simulink model "factMatWhile"  (R2016b)
settings: Solver=FixedStepDiscrete  StartTime=0.0  StopTime=10.0  RelTol=1e-3
libraries: simulink x1
settings Model: Creator=Radwa  LastModifiedBy=Radwa
settings SolverCC: EnableConcurrentExecution=on
settings DataIOCC: ReturnWorkspaceOutputs=on
settings OptimizationCC: DefaultParameterBehavior=Inlined  EnhancedBackFolding=on  PassReuseOutputArgsAs=Individual arguments
settings DebuggingCC: ParameterTunabilityLossMsg=error
settings SFSimCC: SimUseLocalCustomCode=on
settings RTWCC: SystemTargetFile=ert.tlc  GenCodeOnly=on  TemplateMakefile=ert_default_tmf  Description=Embedded Coder  GenerateReport=on  RTWUseLocalCustomCode=on  IncludeHyperlinkInReport=on  LaunchReport=on  GenerateTraceInfo=on  GenerateTraceReport=on  GenerateTraceReportSl=on  GenerateTraceReportSf=on  GenerateTraceReportEml=on
settings CodeAppCC: ForceParamTrailComments=on  IgnoreCustomStorageClasses=off  OperatorAnnotations=on  SimulinkDataObjDesc=on  SFDataObjDesc=on  InsertBlockDesc=on
settings ERTTargetCC: TargetLangStandard=C99 (ISO)  MultiwordLength=256  GenerateSampleERTMain=on  InlinedParameterPlacement=NonHierarchical  ERTCustomFileTemplate=example_file_process.tlc

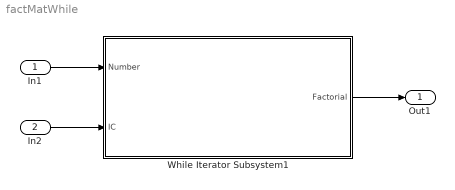
== system factMatWhile ==
  In1 : Inport
  In2 : Inport  Port=2
  While Iterator Subsystem1 : Subsystem  TreatAsAtomicUnit=on
  Out1 : Outport
  wires:
  In1/1 -> While Iterator Subsystem1/1(Number)
  While Iterator Subsystem1/1(Factorial) -> Out1/1
  In2/1 -> While Iterator Subsystem1/2(IC)

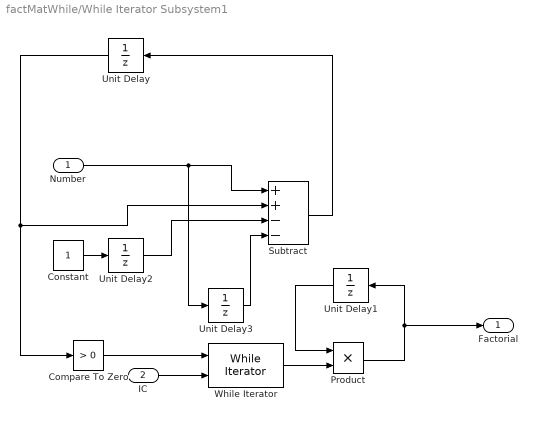
== system factMatWhile/While Iterator Subsystem1 ==
  Number : Inport
  IC : Inport  Port=2
  Compare To Zero : simulink/Logic and Bit Operations/Compare To Zero  relop=>  OutDataTypeStr=boolean
  Constant : Constant
  Product : Product
  Subtract : Sum  Inputs=++--
  Unit Delay : UnitDelay  SampleTime=-1
  Unit Delay1 : UnitDelay  InitialCondition=1  SampleTime=-1
  Unit Delay2 : UnitDelay  SampleTime=-1
  Unit Delay3 : UnitDelay  SampleTime=-1
  While Iterator : WhileIterator  MaxIters=6  ShowIterationPort=on  OutputDataType=double
  Factorial : Outport
  wires:
  IC/1 -> While Iterator/2
  Subtract/1 -> Unit Delay/1
  While Iterator/1 -> Product/2
  Product/1 -> Factorial/1, Unit Delay1/1
  Unit Delay1/1 -> Product/1
  Constant/1 -> Unit Delay2/1
  Unit Delay2/1 -> Subtract/3
  Number/1 -> Subtract/1, Unit Delay3/1
  Compare To Zero/1 -> While Iterator/1
  Unit Delay/1 -> Compare To Zero/1, Subtract/2
  Unit Delay3/1 -> Subtract/4
